simulink subsystem "rss_SplyVltgLoLvl2Dia"  (R2023a)
settings: Solver=VariableStepAuto  StartTime=0.0  StopTime=10.0  RelTol=1e-3
undefined symbols (not defined in the file): Cdbl_uSplyVltgMaxVal, ENM_TYPE_FALT, Gu16_ctSplyVltgLoLvl2ConfCnt_C, Gu16_ctSplyVltgLoLvl2RcvyCnt_C, Gu16_uSplyVltgLoLvl2ConfTrs_C, Gu16_uSplyVltgLoLvl2RcvyTrs_C
libraries: vhit_control_library x1, lib_fault_definiteness x1
settings Model: Creator=xiaoqiang.yuan  LastModifiedBy=xiaoqiang.yuan

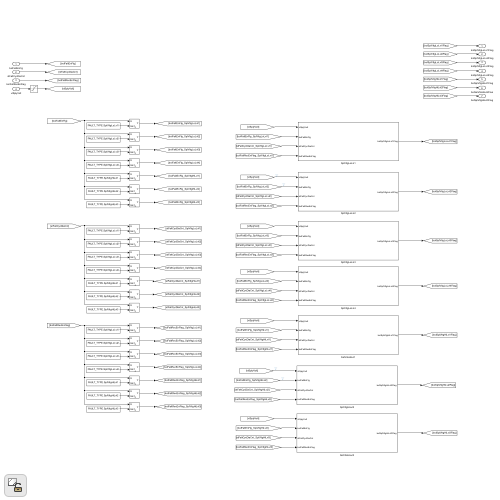
[thumbnail: Simulink's stored preview of the top-level diagram]
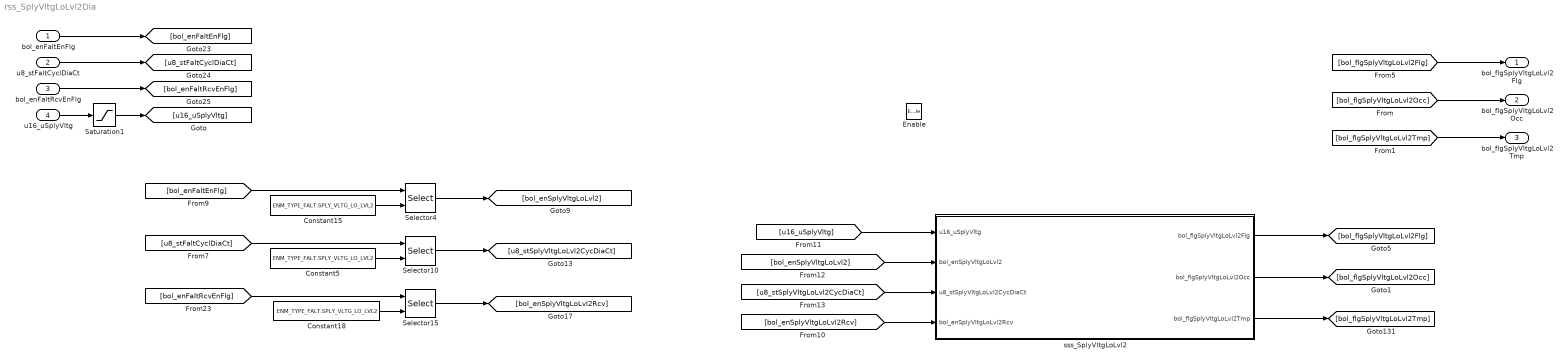
== system rss_SplyVltgLoLvl2Dia ==
  bol_enFaltEnFlg : Inport  OutDataTypeStr=boolean
  u8_stFaltCyclDiaCt : Inport  Port=2  OutDataTypeStr=uint8
  bol_enFaltRcvEnFlg : Inport  Port=3  OutDataTypeStr=boolean
  u16_uSplyVltg : Inport  Port=4  OutDataTypeStr=dt_Standardize_u16p15b0
  Enable : EnablePort
  Constant15 : Constant  Value=ENM_TYPE_FALT.SPLY_VLTG_LO_LVL2
  Constant18 : Constant  Value=ENM_TYPE_FALT.SPLY_VLTG_LO_LVL2
  Constant5 : Constant  Value=ENM_TYPE_FALT.SPLY_VLTG_LO_LVL2
  Saturation1 : Saturate  UpperLimit=Cdbl_uSplyVltgMaxVal  LowerLimit=0
  Selector10 : Selector  IndexMode=Zero-based  InputPortWidth=Cdbl_numFaltDiaNum  IndexOptions=Index vector (port)  Indices=[1 3]  OutputSizes=1
  Selector15 : Selector  IndexMode=Zero-based  InputPortWidth=Cdbl_numFaltDiaNum  IndexOptions=Index vector (port)  Indices=[1 3]  OutputSizes=1
  Selector4 : Selector  IndexMode=Zero-based  InputPortWidth=Cdbl_numFaltDiaNum  IndexOptions=Index vector (port)  Indices=[1 3]  OutputSizes=1
  sss_SplyVltgLoLvl2 : Subsystem
  bol_flgSplyVltgLoLvl2Flg : Outport  OutDataTypeStr=boolean
  bol_flgSplyVltgLoLvl2Occ : Outport  Port=2  OutDataTypeStr=boolean
  bol_flgSplyVltgLoLvl2Tmp : Outport  Port=3  OutDataTypeStr=boolean
  wires:
  [bol_flgSplyVltgLoLvl2Flg] -> bol_flgSplyVltgLoLvl2Flg/1
  [u16_uSplyVltg] -> sss_SplyVltgLoLvl2/1(u16_uSplyVltg)
  [bol_enSplyVltgLoLvl2] -> sss_SplyVltgLoLvl2/2(bol_enSplyVltgLoLvl2)
  Selector4/1 -> [bol_enSplyVltgLoLvl2]
  [u8_stSplyVltgLoLvl2CycDiaCt] -> sss_SplyVltgLoLvl2/3(u8_stSplyVltgLoLvl2CycDiaCt)
  sss_SplyVltgLoLvl2/1(bol_flgSplyVltgLoLvl2Flg) -> [bol_flgSplyVltgLoLvl2Flg]
  Constant15/1 -> Selector4/2
  [bol_enSplyVltgLoLvl2Rcv] -> sss_SplyVltgLoLvl2/4(bol_enSplyVltgLoLvl2Rcv)
  [bol_enFaltEnFlg] -> Selector4/1
  bol_enFaltEnFlg/1 -> [bol_enFaltEnFlg]
  bol_enFaltRcvEnFlg/1 -> [bol_enFaltRcvEnFlg]
  u8_stFaltCyclDiaCt/1 -> [u8_stFaltCyclDiaCt]
  Selector10/1 -> [u8_stSplyVltgLoLvl2CycDiaCt]
  [u8_stFaltCyclDiaCt] -> Selector10/1
  Selector15/1 -> [bol_enSplyVltgLoLvl2Rcv]
  u16_uSplyVltg/1 -> Saturation1/1
  Saturation1/1 -> [u16_uSplyVltg]
  Constant5/1 -> Selector10/2
  Constant18/1 -> Selector15/2
  [bol_enFaltRcvEnFlg] -> Selector15/1
  sss_SplyVltgLoLvl2/2(bol_flgSplyVltgLoLvl2Occ) -> [bol_flgSplyVltgLoLvl2Occ]
  [bol_flgSplyVltgLoLvl2Occ] -> bol_flgSplyVltgLoLvl2Occ/1
  [bol_flgSplyVltgLoLvl2Tmp] -> bol_flgSplyVltgLoLvl2Tmp/1
  sss_SplyVltgLoLvl2/3(bol_flgSplyVltgLoLvl2Tmp) -> [bol_flgSplyVltgLoLvl2Tmp]

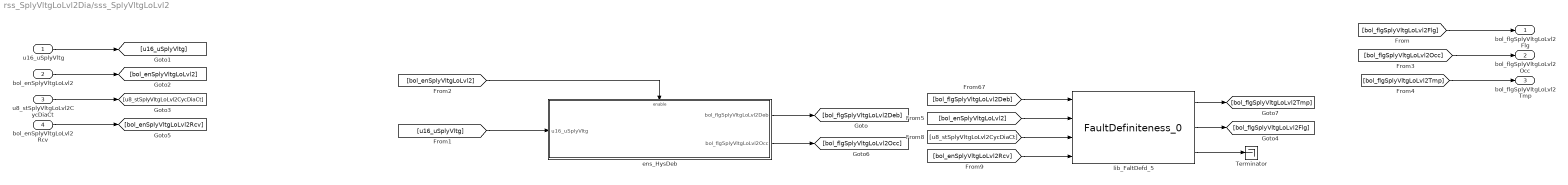
== system rss_SplyVltgLoLvl2Dia/sss_SplyVltgLoLvl2 ==
  u16_uSplyVltg : Inport
  bol_enSplyVltgLoLvl2 : Inport  Port=2
  u8_stSplyVltgLoLvl2CycDiaCt : Inport  Port=3
  bol_enSplyVltgLoLvl2Rcv : Inport  Port=4
  Terminator : Terminator
  ens_HysDeb : Subsystem
  lib_FaltDefd_5 : lib_fault_definiteness/FaultDefiniteness_0  lb_FaltWaitRecvCnt=Gu16_ctSplyVltgLoLvl2ConfCnt_C
  bol_flgSplyVltgLoLvl2Flg : Outport
  bol_flgSplyVltgLoLvl2Occ : Outport  Port=2
  bol_flgSplyVltgLoLvl2Tmp : Outport  Port=3
  wires:
  [bol_flgSplyVltgLoLvl2Tmp] -> bol_flgSplyVltgLoLvl2Tmp/1
  [bol_flgSplyVltgLoLvl2Occ] -> bol_flgSplyVltgLoLvl2Occ/1
  ens_HysDeb/2(bol_flgSplyVltgLoLvl2Occ) -> [bol_flgSplyVltgLoLvl2Occ]
  lib_FaltDefd_5/1 -> [bol_flgSplyVltgLoLvl2Tmp]
  lib_FaltDefd_5/2 -> [bol_flgSplyVltgLoLvl2Flg]
  lib_FaltDefd_5/3 -> Terminator/1
  [bol_flgSplyVltgLoLvl2Deb] -> lib_FaltDefd_5/1
  [bol_enSplyVltgLoLvl2] -> lib_FaltDefd_5/2
  [u8_stSplyVltgLoLvl2CycDiaCt] -> lib_FaltDefd_5/3
  [bol_enSplyVltgLoLvl2Rcv] -> lib_FaltDefd_5/4
  u16_uSplyVltg/1 -> [u16_uSplyVltg]
  [bol_flgSplyVltgLoLvl2Flg] -> bol_flgSplyVltgLoLvl2Flg/1
  bol_enSplyVltgLoLvl2/1 -> [bol_enSplyVltgLoLvl2]
  u8_stSplyVltgLoLvl2CycDiaCt/1 -> [u8_stSplyVltgLoLvl2CycDiaCt]
  bol_enSplyVltgLoLvl2Rcv/1 -> [bol_enSplyVltgLoLvl2Rcv]
  ens_HysDeb/1(bol_flgSplyVltgLoLvl2Deb) -> [bol_flgSplyVltgLoLvl2Deb]
  [u16_uSplyVltg] -> ens_HysDeb/1(u16_uSplyVltg)
  [bol_enSplyVltgLoLvl2] -> ens_HysDeb/Enable

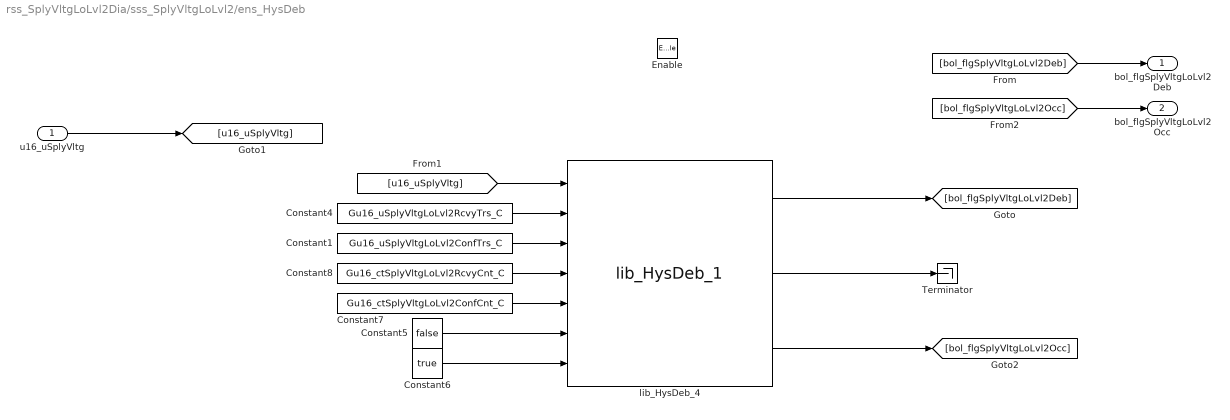
== system rss_SplyVltgLoLvl2Dia/sss_SplyVltgLoLvl2/ens_HysDeb ==
  u16_uSplyVltg : Inport
  Enable : EnablePort
  Constant1 : Constant  Value=Gu16_uSplyVltgLoLvl2ConfTrs_C
  Constant4 : Constant  Value=Gu16_uSplyVltgLoLvl2RcvyTrs_C
  Constant5 : Constant  Value=false  OutDataTypeStr=boolean
  Constant6 : Constant  Value=true  OutDataTypeStr=boolean
  Constant7 : Constant  Value=Gu16_ctSplyVltgLoLvl2ConfCnt_C
  Constant8 : Constant  Value=Gu16_ctSplyVltgLoLvl2RcvyCnt_C
  Terminator : Terminator
  lib_HysDeb_4 : vhit_control_library/lib_HysDeb_1  lb_parInitOutp=0
  bol_flgSplyVltgLoLvl2Deb : Outport
  bol_flgSplyVltgLoLvl2Occ : Outport  Port=2
  wires:
  [bol_flgSplyVltgLoLvl2Occ] -> bol_flgSplyVltgLoLvl2Occ/1
  lib_HysDeb_4/3 -> [bol_flgSplyVltgLoLvl2Occ]
  lib_HysDeb_4/2 -> Terminator/1
  Constant1/1 -> lib_HysDeb_4/3
  Constant4/1 -> lib_HysDeb_4/2
  Constant8/1 -> lib_HysDeb_4/4
  Constant7/1 -> lib_HysDeb_4/5
  lib_HysDeb_4/1 -> [bol_flgSplyVltgLoLvl2Deb]
  Constant6/1 -> lib_HysDeb_4/7
  Constant5/1 -> lib_HysDeb_4/6
  [u16_uSplyVltg] -> lib_HysDeb_4/1
  [bol_flgSplyVltgLoLvl2Deb] -> bol_flgSplyVltgLoLvl2Deb/1
  u16_uSplyVltg/1 -> [u16_uSplyVltg]
